simulink model "mass_spring_damper"  (R2019b)
settings: Solver=VariableStepAuto  StartTime=0.0  StopTime=10  RelTol=1e-3
model workspace (MAT data in the model file):
  J = Simulink.Parameter
  J.Value = 1
  J.DataType = 'auto'
  J.Dimensions = [1 1]
  b = Simulink.Parameter
  b.Value = 10
  b.DataType = 'auto'
  b.Dimensions = [1 1]
  k = Simulink.Parameter
  k.Value = 5
  k.DataType = 'auto'
  k.Dimensions = [1 1]
  theta_0 = 0
undefined symbols (not defined in the file): NULL, serial
libraries: instrumentlib x3
settings Model: OrderedModelArguments=off  Creator=mackenziegray  LastModifiedBy=mackenziegray
settings DataIOCC: ExternalInput=[theta_0, theta00]

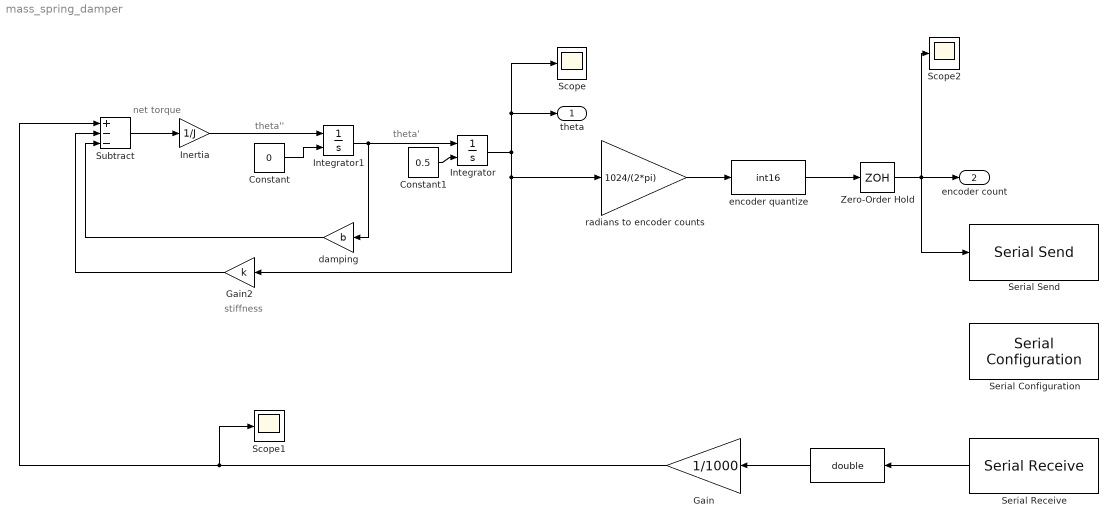
== system mass_spring_damper ==
  note: theta'
  note: theta''
  note: net torque
  note: stiffness
  " " : DataTypeConversion  OutDataTypeStr=double
  Constant : Constant  Value=0
  Constant1 : Constant  Value=0.5
  Gain : Gain  Gain=1/1000
  Gain2 : Gain  Gain=k
  Inertia : Gain  Gain=1/J
  Integrator : Integrator  InitialConditionSource=external  InitialCondition=theta_0
  Integrator1 : Integrator  InitialConditionSource=external
  Scope : Scope
  Scope1 : Scope
  Scope2 : Scope
  Serial Configuration : instrumentlib/Serial Configuration  Priority=-200000  ComPortMenu=/dev/tty.usbmodem0E23029F1  ComPort=/dev/tty.usbmodem0E23029F1  ObjConstructor=serial('/dev/tty.usbmodem0E23029F1');  BaudRate=115200  DataBits=8  Parity=none  StopBits=1  FlowControl=none  Timeout=10  ByteOrder=LittleEndian
  Serial Receive : instrumentlib/Serial Receive  ComPortMenu=/dev/tty.usbmodem0E23029F1  ComPort=/dev/tty.usbmodem0E23029F1  ObjConstructor=serial('/dev/tty.usbmodem0E23029F1');  Terminator=NULL ('\0')  DataSize=[1 1]  DataType=int16  EnableBlockingMode=on  ActionDataUnavailable=Output last received value  CustomValue=0  SampleTime=.1
  Serial Send : instrumentlib/Serial Send  ComPortMenu=/dev/tty.usbmodem0E23029F1  ComPort=/dev/tty.usbmodem0E23029F1  ObjConstructor=serial('/dev/tty.usbmodem0E23029F1');  Terminator=NULL ('\0')  EnableBlockingMode=on
  Subtract : Sum  Inputs=+--
  Zero-Order Hold : ZeroOrderHold  SampleTime=-1
  damping : Gain  Gain=b
  encoder quantize : DataTypeConversion  OutDataTypeStr=int16
  radians to encoder counts : Gain  Gain=1024/(2*pi)
  theta : Outport
  encoder count : Outport  Port=2
  wires:
  Inertia/1 -> Integrator1/1
  Integrator1/1 -> damping/1, Integrator/1
  damping/1 -> Subtract/3
  Subtract/1 -> Inertia/1
  Integrator/1 -> radians to encoder counts/1, Gain2/1, theta/1, Scope/1
  radians to encoder counts/1 -> encoder quantize/1
  encoder quantize/1 -> Zero-Order Hold/1
  Zero-Order Hold/1 -> Scope2/1, encoder count/1, Serial Send/1
  Serial Receive/1 -> " "/1
  " "/1 -> Gain/1
  Gain/1 -> Subtract/1, Scope1/1
  Gain2/1 -> Subtract/2
  Constant/1 -> Integrator1/2
  Constant1/1 -> Integrator/2
